simulink model "ES200A_CurrMeas"  (R2013b)
settings: Solver=FixedStepDiscrete  SolverMode=SingleTasking  StartTime=0.0  StopTime=1  FixedStep=0.000125  RelTol=1e-3
undefined symbols (not defined in the file): ARCHGLBPRM_2PI_ULS_F32, CurrMeasEolGainMax, CurrMeasEolGainMin, CurrMeasEolGainNrOfSample, CurrMeasEolGainNumer, CurrMeasEolMaxMotVel, CurrMeasEolOffsHiBrdgVltgMin, CurrMeasEolOffsHiCmuOffs, CurrMeasEolOffsLoCmuOffs, CurrMeasEolOffsMax, CurrMeasEolOffsMin, CurrMeasEolOffsNrOfSample, CurrMeasEolTranCntrThd, CurrMeasMinRqrdPhaOnTi, CurrMeasMotAgCompuDly, CurrMeasMotCurrAdcVlyWrmIninMax, CurrMeasMotCurrAdcVlyWrmIninMin, CurrMeasNtc0x05DFailStep, CurrMeasNtc0x05DPassStep, CurrMeasNtc0x06DFailStep, CurrMeasNtc0x06DPassStep, DEGREES30_MOTRAD_F32, DIFOFFSRNGCHKMAX_VOLT_F32, ELECGLBPRM_IVTRCNT_CNT_U08, ELECGLBPRM_STRTUPSTCURRMEASWRMININTESTSTRT_CNT_U08, FLTINJ_CURRMEAS_MOTCURRCORRDA, FLTINJ_CURRMEAS_MOTCURRCORRDD, FLTINJ_CURRMEAS_TESTOK, MAXCURRCORRD_AMPR_F32, PhaABCMeasdOutOfRng, PhaDEFMeasOutOfRng, SysGlbPrmMotPoleCnt
libraries: simulink x10, FixdToFloat x1
(part 7 of 7)

== stateflow chart ES200A_CurrMeas/CurrMeas/CurrMeasPer1/Offset Calibration/Offset State Machine ==
  note: EolOffsSts
      |
      | 0 = Not Started
      | 1 = Started/In Process
      | 2 = Successful
      | 4  = Phase A, B, C EOL Calculated Gains are Out Of Range
      | 8  = Phase D, E, F EOL Calculated Gains are Out Of Range
      | 12 = Phase A, B, C, D, E, F EOL Calculated Gains are Out Of Range
      | 16  = VehSpd, VehSpdVld, condition not met
      | 32  = MotVelMrf condition not met
      | 64 = DiagcStsIvtr1Inactv and DiagcStsIvtr1Inactv both TRUE
  note: EolOffsOutOfRng = NTCNR_0X1EC
      | Parameters:
      |        Bit0Descr = 1 = 0000 0001 = Phase A, B, C EOL Calculated Offsets are Out Of Range
      |        Bit1Descr = 2 = 0000 0010 = Phase D, E, F EOL Calculated Offsets are Out Of Range
      |        Bit0Descr | Bit1Descr = 3 = 0000 0011 = Phase A, B, C, D, E, F EOL Calculated Offsets are Out Of Range
      |        Bit2Descr = 4 = 0000 0100 = VehSpd, VehSpdVld, condition not met
      |        Bit3Descr = 8 = 0000 1000 = MotVelMrf condition not met
      |        Bit3Descr = 16 = 0001 0000 = DiagcStsIvtr1Inactv and DiagcStsIvtr1Inactv both TRUE
  note: ***Rev 4.6.0 Change***
      | Replace:
      | {OffsRngChkABC = 1;}
      |
      | With:
      | {OffsRngChkABC = 0;}
      | **************************
  note: ***Rev 4.6.0 Change***
      | Replace:
      | {OffsRngChkDEF = 1;}
      |
      | With:
      | {OffsRngChkDEF = 0;}
      | **************************
  state MotCurrNtcSet = SetNtcSts(NTCNr,ParamBit,NTCSts,NTCDebStep) [function]
  note: EolOffsSts
      |
      | 0 = Not Started
      | 1 = Started/In Process
      | 2 = Successful
      | 4  = Phase A, B, C EOL Calculated Gains are Out Of Range
      | 8  = Phase D, E, F EOL Calculated Gains are Out Of Range
      | 12 = Phase A, B, C, D, E, F EOL Calculated Gains are Out Of Range
      | 16  = VehSpd, VehSpdVld, condition not met
      | 32  = MotVelMrf condition not met
      | 64 = DiagcStsIvtr1Inactv and DiagcStsIvtr1Inactv both TRUE
  note: EolOffsOutOfRng = NTCNR_0X1EC
      | Parameters:
      |        Bit0Descr = 1 = 0000 0001 = Phase A, B, C EOL Calculated Offsets are Out Of Range
      |        Bit1Descr = 2 = 0000 0010 = Phase D, E, F EOL Calculated Offsets are Out Of Range
      |
      |        Bit0Descr | Bit1Descr = 3 = 0000 0011 = Phase A, B, C, D, E, F EOL Calculated Offsets are Out Of Range
      |
      |        Bit2Descr = 4 = 0000 0100 = VehSpd, VehSpdVld, condition not met
      |        Bit3Descr = 8 = 0000 1000 = MotVelMrf condition not met
      |        Bit3Descr = 16 = 0001 0000 = DiagcStsIvtr1Inactv and DiagcStsIvtr1Inactv both TRUE
  state WrNvm [function]
  (default) -> (junction 307) : {EolOffsSts = EolOffsStsPrev;}
  (junction 307) -> (junction 233) [order 2] : {EolOffsSts = EolOffsStsPrev;}
  (junction 307) -> (junction 188) [order 1] : [EolOffsSts == 1]
  (junction 188) -> (junction 452) [order 1] : [(VehSpd <= ARCHGLBPRM_FLOATZEROTHD_ULS_F32 )...
      |  && (VehSpdVld == 1)]
  (junction 452) -> (junction 186) [order 1] : [(abs(MotVelMrf) <= CurrMeasEolMaxMotVel)]
  (junction 186) -> (junction 245) [order 2]
  (junction 245) -> (junction 263) [order 2]
  (junction 263) -> (junction 284) [order 2]
  (junction 284) -> (junction 294) [order 2]
  (junction 452) -> (junction 455) [order 2] : {CurrMeasMotCurrEolCalSt = MotCurrEolCalSt2.MCECS_CMDSAFEST;
      | MotCurrNtcSet = SetNtcSts(EolOffsOutOfRng, 8, 1, 0);
      | EolOffsSts = 32;}
  (junction 188) -> (junction 233) [order 2] : {CurrMeasMotCurrEolCalSt = MotCurrEolCalSt2.MCECS_CMDSAFEST;
      | MotCurrNtcSet = SetNtcSts(EolOffsOutOfRng, 4, 1, 0);
      | EolOffsSts = 16;}
  (junction 186) -> (junction 194) [order 1] : [(CurrMeasMotCurrEolCalStPrev == 0) || (CurrMeasMotCurrEolCalStPrev == 1)]
      | {CurrMeasMotCurrEolCalSt = MotCurrEolCalSt2.MCECS_OFFSCMDHI;}
  (junction 245) -> (junction 238) [order 1] : [CurrMeasMotCurrEolCalStPrev == MotCurrEolCalSt2.MCECS_OFFSCMDLO]
  (junction 263) -> (junction 256) [order 1] : [CurrMeasMotCurrEolCalStPrev == MotCurrEolCalSt2.MCECS_OFFSCMDZERO]
  (junction 284) -> (junction 395) [order 1] : [CurrMeasMotCurrEolCalStPrev == MotCurrEolCalSt2.MCECS_OFFSCMDEND && MotCurrEolOffsProcFlg != 1]
  (junction 294) -> (junction 295)
  (junction 395) -> (junction 414) [order 2] : {OffsRngChkABC = 0;}
  (junction 395) -> (junction 281) [order 1] : [DiagcStsIvtr1Inactv == 0]
  (junction 281) -> (junction 418) [order 2]
  (junction 418) -> (junction 434) : {OffsFltParam = 1;
      | OffsRngChkABC = 0;}
  (junction 281) -> (junction 414) [order 1] : [((MotCurrOffsHiAvrgA >= CurrMeasEolOffsMin) && (MotCurrOffsHiAvrgA <= CurrMeasEolOffsMax)) &&...
      | ((MotCurrOffsHiAvrgB >= CurrMeasEolOffsMin) && (MotCurrOffsHiAvrgB <= CurrMeasEolOffsMax)) &&...
      | ((MotCurrOffsHiAvrgC >= CurrMeasEolOffsMin) && (MotCurrOffsHiAvrgC <= CurrMeasEolOffsMax)) &&...
      | ((MotCurrOffsLoAvrgA >= CurrMeasEolOffsMin) && (MotCurrOffsLoAvrgA <= CurrMeasEolOffsMax)) &&...
      | ((MotCurrOffsLoAvrgB >= CurrMeasEolOffsMin) && (MotCurrOffsLoAvrgB <= CurrMeasEolOffsMax)) &&...
      | ((MotCurrOffsLoAvrgC >= CurrMeasEolOffsMin) && (MotCurrOffsLoAvrgC <= CurrMeasEolOffsMax))]
      |
      | {OffsRngChkABC = 1;}
  (junction 194) -> (junction 204) [order 2] : {CurrMeasEolTranCntr = CurrMeasEolTranCntrPrev + 1;}
  (junction 238) -> (junction 249) [order 2] : {CurrMeasEolTranCntr = CurrMeasEolTranCntrPrev + 1;}
  (junction 256) -> (junction 261) [order 2] : {CurrMeasEolTranCntr = CurrMeasEolTranCntrPrev + 1;}
  (junction 194) -> (junction 200) [order 1] : [CurrMeasEolTranCntr == CurrMeasEolTranCntrThd]
      |
      | {CurrMeasMotCurrSumA = CurrMeasMotCurrSumAPrev + MotCurrAdcVlyA;
      | CurrMeasMotCurrSumB = CurrMeasMotCurrSumBPrev + MotCurrAdcVlyB;
      | CurrMeasMotCurrSumC = CurrMeasMotCurrSumCPrev + MotCurrAdcVlyC;
      | CurrMeasMotCurrSumD = CurrMeasMotCurrSumDPrev + MotCurrAdcVlyD;
      | CurrMeasMotCurrSumE = CurrMeasMotCurrSumEPrev + MotCurrAdcVlyE;
      | CurrMeasMotCurrSumF = CurrMeasMotCurrSumFPrev + MotCurrAdcVlyF;
      | CurrMeasBrdgVltgSum = CurrMeasBrdgVltgSumPrev + BrdgVltg;
      |
      | CurrMeasEolAvrgCntr = CurrMeasEolAvrgCntrPrev + 1;}
  (junction 238) -> (junction 241) [order 1] : [CurrMeasEolTranCntr == CurrMeasEolTranCntrThd]
      |
      | {CurrMeasMotCurrSumA = CurrMeasMotCurrSumAPrev + MotCurrAdcVlyA;
      | CurrMeasMotCurrSumB = CurrMeasMotCurrSumBPrev + MotCurrAdcVlyB;
      | CurrMeasMotCurrSumC = CurrMeasMotCurrSumCPrev + MotCurrAdcVlyC;
      | CurrMeasMotCurrSumD = CurrMeasMotCurrSumDPrev + MotCurrAdcVlyD;
      | CurrMeasMotCurrSumE = CurrMeasMotCurrSumEPrev + MotCurrAdcVlyE;
      | CurrMeasMotCurrSumF = CurrMeasMotCurrSumFPrev + MotCurrAdcVlyF;
      |
      |
      | CurrMeasEolAvrgCntr = CurrMeasEolAvrgCntrPrev + 1;}
  (junction 256) -> (junction 254) [order 1] : [CurrMeasEolTranCntr == CurrMeasEolTranCntrThd]
      |
      | {CurrMeasMotCurrSumA = CurrMeasMotCurrSumAPrev + MotCurrAdcVlyA;
      | CurrMeasMotCurrSumB = CurrMeasMotCurrSumBPrev + MotCurrAdcVlyB;
      | CurrMeasMotCurrSumC = CurrMeasMotCurrSumCPrev + MotCurrAdcVlyC;
      | CurrMeasMotCurrSumD = CurrMeasMotCurrSumDPrev + MotCurrAdcVlyD;
      | CurrMeasMotCurrSumE = CurrMeasMotCurrSumEPrev + MotCurrAdcVlyE;
      | CurrMeasMotCurrSumF = CurrMeasMotCurrSumFPrev + MotCurrAdcVlyF;
      |
      |
      | CurrMeasEolAvrgCntr = CurrMeasEolAvrgCntrPrev + 1;}
  (junction 434) -> (junction 414)
  (junction 414) -> (junction 368)
  (junction 368) -> (junction 283) [order 2] : {OffsRngChkDEF = 0;}
  (junction 368) -> (junction 398) [order 1] : [DiagcStsIvtr2Inactv == 0 && ELECGLBPRM_IVTRCNT_CNT_U08 == 2]
  (junction 398) -> (junction 421) [order 2]
  (junction 421) -> (junction 436) : {OffsFltParam = OffsFltParam + 2
      | OffsRngChkDEF = 0;}
  (junction 398) -> (junction 283) [order 1] : [((MotCurrOffsHiAvrgD >= CurrMeasEolOffsMin) && (MotCurrOffsHiAvrgD <= CurrMeasEolOffsMax)) &&...
      | ((MotCurrOffsHiAvrgE >= CurrMeasEolOffsMin) && (MotCurrOffsHiAvrgE <= CurrMeasEolOffsMax)) &&...
      | ((MotCurrOffsHiAvrgF >= CurrMeasEolOffsMin) && (MotCurrOffsHiAvrgF <= CurrMeasEolOffsMax)) &&...
      | ((MotCurrOffsLoAvrgD >= CurrMeasEolOffsMin) && (MotCurrOffsLoAvrgD <= CurrMeasEolOffsMax)) &&...
      | ((MotCurrOffsLoAvrgE >= CurrMeasEolOffsMin) && (MotCurrOffsLoAvrgE <= CurrMeasEolOffsMax)) &&...
      | ((MotCurrOffsLoAvrgF >= CurrMeasEolOffsMin) && (MotCurrOffsLoAvrgF <= CurrMeasEolOffsMax))]
      |
      | {OffsRngChkDEF = 1;}
  (junction 436) -> (junction 283)
  (junction 283) -> (junction 439)
  (junction 200) -> (junction 204) [order 2]
  (junction 241) -> (junction 249) [order 2]
  (junction 254) -> (junction 261) [order 2]
  (junction 200) -> (junction 204) [order 1] : [CurrMeasEolAvrgCntr == CurrMeasEolOffsNrOfSample]
      |
      | {MotCurrOffsHiAvrgA = CurrMeasMotCurrSumA / CurrMeasEolOffsNrOfSample;
      | MotCurrOffsHiAvrgB = CurrMeasMotCurrSumB / CurrMeasEolOffsNrOfSample;
      | MotCurrOffsHiAvrgC = CurrMeasMotCurrSumC / CurrMeasEolOffsNrOfSample;
      | MotCurrOffsHiAvrgD = CurrMeasMotCurrSumD / CurrMeasEolOffsNrOfSample;
      | MotCurrOffsHiAvrgE = CurrMeasMotCurrSumE / CurrMeasEolOffsNrOfSample;
      | MotCurrOffsHiAvrgF = CurrMeasMotCurrSumF / CurrMeasEolOffsNrOfSample;
      | BrdgVltgAvrg  = CurrMeasBrdgVltgSum / CurrMeasEolOffsNrOfSample;
      | MotCurrEolOffsHiBrdgVltg = BrdgVltgAvrg * (CurrMeasEolOffsHiCmuOffs...
      |  - CurrMeasEolOffsLoCmuOffs);
      |
      | CurrMeasMotCurrEolCalSt = MotCurrEolCalSt2.MCECS_OFFSCMDLO;
      |
      | CurrMeasEolAvrgCntr = 0;
      | CurrMeasEolTranCntr = 0;
      |
      | CurrMeasMotCurrSumA = 0;
      | CurrMeasMotCurrSumB = 0;
      | CurrMeasMotCurrSumC = 0;
      | CurrMeasMotCurrSumD = 0;
      | CurrMeasMotCurrSumE = 0;
      | CurrMeasMotCurrSumF = 0;}
  (junction 241) -> (junction 249) [order 1] : [CurrMeasEolAvrgCntr == CurrMeasEolOffsNrOfSample]
      |
      | {MotCurrOffsLoAvrgA = CurrMeasMotCurrSumA / CurrMeasEolOffsNrOfSample;
      | MotCurrOffsLoAvrgB = CurrMeasMotCurrSumB / CurrMeasEolOffsNrOfSample;
      | MotCurrOffsLoAvrgC = CurrMeasMotCurrSumC / CurrMeasEolOffsNrOfSample;
      | MotCurrOffsLoAvrgD = CurrMeasMotCurrSumD / CurrMeasEolOffsNrOfSample;
      | MotCurrOffsLoAvrgE = CurrMeasMotCurrSumE / CurrMeasEolOffsNrOfSample;
      | MotCurrOffsLoAvrgF = CurrMeasMotCurrSumF / CurrMeasEolOffsNrOfSample;
      |
      |
      |
      |
      | CurrMeasMotCurrEolCalSt = MotCurrEolCalSt2.MCECS_OFFSCMDZERO;
      |
      | CurrMeasEolAvrgCntr = 0;
      | CurrMeasEolTranCntr = 0;
      |
      | CurrMeasMotCurrSumA = 0;
      | CurrMeasMotCurrSumB = 0;
      | CurrMeasMotCurrSumC = 0;
      | CurrMeasMotCurrSumD = 0;
      | CurrMeasMotCurrSumE = 0;
      | CurrMeasMotCurrSumF = 0;}
  (junction 254) -> (junction 261) [order 1] : [CurrMeasEolAvrgCntr == CurrMeasEolOffsNrOfSample]
      |
      | {MotCurrOffsZeroAvrgA = CurrMeasMotCurrSumA / CurrMeasEolOffsNrOfSample;
      | MotCurrOffsZeroAvrgB = CurrMeasMotCurrSumB / CurrMeasEolOffsNrOfSample;
      | MotCurrOffsZeroAvrgC = CurrMeasMotCurrSumC / CurrMeasEolOffsNrOfSample;
      | MotCurrOffsZeroAvrgD = CurrMeasMotCurrSumD / CurrMeasEolOffsNrOfSample;
      | MotCurrOffsZeroAvrgE = CurrMeasMotCurrSumE / CurrMeasEolOffsNrOfSample;
      | MotCurrOffsZeroAvrgF = CurrMeasMotCurrSumF / CurrMeasEolOffsNrOfSample;
      |
      |
      |
      |
      | CurrMeasMotCurrEolCalSt = MotCurrEolCalSt2.MCECS_OFFSCMDEND;
      |
      | CurrMeasEolAvrgCntr = 0;
      | CurrMeasEolTranCntr = 0;
      |
      | CurrMeasMotCurrSumA = 0;
      | CurrMeasMotCurrSumB = 0;
      | CurrMeasMotCurrSumC = 0;
      | CurrMeasMotCurrSumD = 0;
      | CurrMeasMotCurrSumE = 0;
      | CurrMeasMotCurrSumF = 0;}
  (junction 439) -> (junction 441) [order 2]
  (junction 441) -> (junction 417) : {
      | CurrMeasMotCurrEolCalSt = MotCurrEolCalSt2.MCECS_CMDSAFEST
      | MotCurrNtcSet = SetNtcSts(EolOffsOutOfRng, OffsFltParam, 1, 0);
      | EolOffsSts = OffsFltParam * 4;
      | CurrMeasEolAvrgCntr = 0;
      | CurrMeasEolTranCntr = 0;
      | }
  (junction 439) -> (junction 443) [order 1] : [OffsRngChkABC == 1 && OffsRngChkDEF == 1]
      | {
      | CurrMeasMotCurrEolCalSt = MotCurrEolCalSt2.MCECS_OFFSCMDEND;
      | CurrMeasEolAvrgCntr = 0;
      | CurrMeasEolTranCntr = 0;
      | }
  (junction 443) -> (junction 445) [order 2]
  (junction 445) -> (junction 422) : {
      | MotCurrNtcSet = SetNtcSts(EolOffsOutOfRng, 16, 1, 0);
      | EolOffsSts = 64;
      | CurrMeasMotCurrEolCalSt = MotCurrEolCalSt2.MCECS_CMDSAFEST;
      | }
  (junction 443) -> (junction 288) [order 1] : [(DiagcStsIvtr1Inactv == 0 || DiagcStsIvtr2Inactv == 0)]
      | {
      | MotCurrNtcSet = SetNtcSts(EolOffsOutOfRng, 0, 0, 0);
      | WrNvm();
      | MotCurrEolOffsProcFlg = 1;
      | EolOffsSts = 2;
      | }
  (junction 233) -> (junction 455)
  (junction 455) -> (junction 204)
  (junction 204) -> (junction 249)
  (junction 249) -> (junction 261)
  (junction 261) -> (junction 417)
  (junction 417) -> (junction 422)
  (junction 422) -> (junction 288)
  (junction 295) -> (junction 288)
  (junction 288) -> (junction 428)
  data: NTCNr function_input; ParamBit function_input; MotCurrNtcSet function_output; NTCSts function_input; NTCDebStep function_input; CurrMeasMotCurrEolCalSt output Enum: MotCurrEolCalSt2; EolOffsSts output uint8; MotCurrAdcVlyA input; MotCurrAdcVlyB input; MotCurrAdcVlyC input; MotCurrAdcVlyD input; MotCurrAdcVlyE input; MotCurrAdcVlyF input; BrdgVltg input; CurrMeasEolOffsNrOfSample input; CurrMeasEolOffsHiCmuOffs input; CurrMeasEolOffsLoCmuOffs input; CurrMeasEolOffsMax input; CurrMeasEolOffsMin input; BrdgVltgAvrg local double; BrdgVltgSum local double; MotCurrOffAvrgCntr local single; MotCurrSumHiA local single; MotCurrSumHiB local single; MotCurrSumHiC local single; MotCurrSumLoA local single; MotCurrSumLoB local single; MotCurrSumLoC local single; MotCurrSumZeroA local single; MotCurrSumZeroB local single; MotCurrSumZeroC local single; MotCurrOffsZeroAvrgA output single; MotCurrOffsZeroAvrgB output single; MotCurrOffsZeroAvrgC output single; MotCurrOffsZeroAvrgD output single; MotCurrOffsZeroAvrgE output single; MotCurrOffsZeroAvrgF output single; MotCurrEolOffsProcFlg output boolean; MotCurrEolOffsHiBrdgVltg output single; MotCurrOffsHiAvrgA output single; MotCurrOffsHiAvrgB output single; MotCurrOffsHiAvrgC output single; MotCurrOffsHiAvrgD output single; MotCurrOffsHiAvrgE output single; MotCurrOffsHiAvrgF output single; MotCurrSumHiD local single; MotCurrSumHiE local single; MotCurrSumHiF local single; MotCurrSumLoD local single; MotCurrSumLoE local single; MotCurrSumLoF local single; MotCurrSumZeroD local single; MotCurrSumZeroE local single; MotCurrSumZeroF local single; MotCurrOffsLoAvrgA output single; MotCurrNtcSet local single; NTC1EC constant single; CurrMeasEolMaxMotVel input; CurrMeasEolTranCntrThd input; MotVelMrf input; VehSpd input; VehSpdVld input; CurrMeasMotCurrEolCalStPrev input; EolOffsStsPrev input; ELECGLBPRM_IVTRCNT_CNT_U08 input; DiagcStsIvtr1Inactv input; DiagcStsIvtr2Inactv input; MotCurrOffsLoAvrgB output single; MotCurrOffsLoAvrgC output single; MotCurrOffsLoAvrgD output single; MotCurrOffsLoAvrgE output single; MotCurrOffsLoAvrgF output single; CurrMeasBrdgVltgSumPrev input; CurrMeasMotCurrSumAPrev input single; CurrMeasMotCurrSumBPrev input; CurrMeasMotCurrSumCPrev input; CurrMeasMotCurrSumDPrev input; CurrMeasMotCurrSumEPrev input; CurrMeasMotCurrSumFPrev input; CurrMeasBrdgVltgSum output single; CurrMeasMotCurrSumA output single; CurrMeasMotCurrSumB output single; CurrMeasMotCurrSumC output single; CurrMeasMotCurrSumD output single; CurrMeasMotCurrSumE output single; CurrMeasMotCurrSumF output single; CurrMeasEolTranCntrPrev input; CurrMeasEolAvrgCntrPrev input; CurrMeasEolTranCntr output uint8; CurrMeasEolAvrgCntr output uint16; EolOffsOutOfRng constant double; OffsRngChkABC local double; OffsRngChkDEF local double; OffsFltParam local double; ARCHGLBPRM_FLOATZEROTHD_ULS_F32 parameter
